simulink model "PPC_navigation_lidar"  (R2026a)
settings: Solver=VariableStepAuto
settings Model: Creator=prana  LastModifiedBy=prana

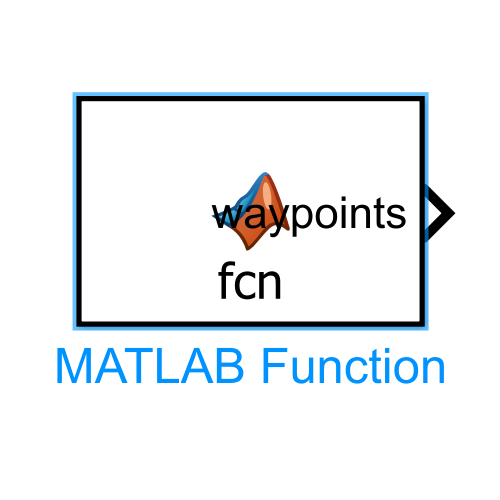
[thumbnail: Simulink's stored preview of the top-level diagram]
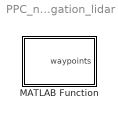
== system PPC_navigation_lidar ==
  MATLAB Function : MATLAB Function  TreatAsAtomicUnit=on

== matlab function PPC_navigation_lidar/MATLAB Function ==
  data: waypoints output
function waypoints = load_waypoints()
    % Output: waypoints - [170 x 4] matrix containing [x, y, z, yaw]
    
    persistent wp_data;
    coder.extrinsic('readmatrix');
    
    if isempty(wp_data)
        % Preallocate matrix dimensions for Simulink signal bus compatibility
        wp_data = zeros(170, 4);
        
        % Read waypoints from text file directly inside the function block
        raw_data = readmatrix('waypoints_3.txt');
        
        num_rows = min(size(raw_data, 1), 170);
        wp_data(1:num_rows, :) = raw_data(1:num_rows, 1:4);
    end
    
    waypoints = wp_data;
end
